simulink model "rcservo1"  (Simulink 7.8)
settings: Solver=ode45  StartTime=0.0  StopTime=10.0  RelTol=1e-3
values from neighbouring files (symbols this model uses):
  atemp = 1e9    (= 1000000000)    [ncf4.m]
libraries: cstblocks x8, simulink x4
settings Model: Creator=kas1d  LastModifiedBy=fukawa
settings DebuggingCC: AlgebraicLoopMsg=none  SolverPrmCheckMsg=none  FcnCallInpInsideContextMsg=Use local settings  UnconnectedInputMsg=none  UnconnectedOutputMsg=none  UnconnectedLineMsg=none

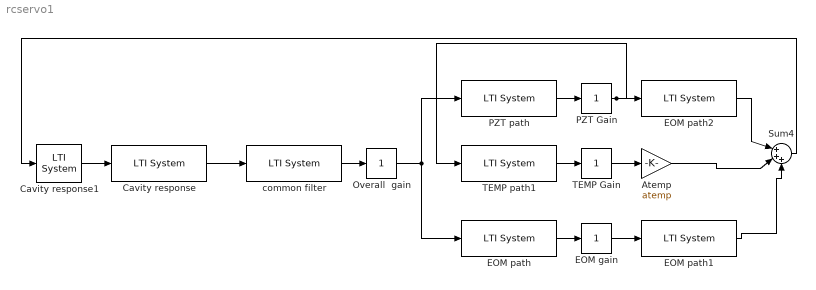
== system rcservo1 ==
  Atemp : Gain  Gain=atemp  SaturateOnIntegerOverflow=on  OutDataTypeStr=Inherit: Same as input  ParamDataTypeStr=Inherit: Same as input
  Cavity response : cstblocks/LTI System  sys=cavity  IC=[0]
  Cavity response1 : cstblocks/LTI System  sys=pmc  IC=[0]
  EOM gain : simulink/Math Operations/Slider Gain  low=0  gain=1  high=2
  EOM path : cstblocks/LTI System  sys=geom  IC=[0]
  EOM path1 : cstblocks/LTI System  sys=aeom  IC=[0]
  EOM path2 : cstblocks/LTI System  sys=apzt  IC=[0]
  Overall  gain : simulink/Math Operations/Slider Gain  low=-1  gain=1  high=2
  PZT Gain : simulink/Math Operations/Slider Gain  low=0  gain=1  high=2
  PZT path : cstblocks/LTI System  sys=gpzt  IC=[0]
  Sum4 : Sum  Inputs=|+++
  TEMP Gain : simulink/Math Operations/Slider Gain  low=0  gain=1  high=2
  TEMP path1 : cstblocks/LTI System  sys=gtemp  IC=[0]
  common filter : cstblocks/LTI System  sys=common  IC=[0]
  wires:
  PZT path/1 -> PZT Gain/1
  PZT Gain/1 -> TEMP path1/1, EOM path2/1
  TEMP Gain/1 -> Atemp/1
  Atemp/1 -> Sum4/2
  TEMP path1/1 -> TEMP Gain/1
  EOM path/1 -> EOM gain/1
  common filter/1 -> Overall  gain/1
  Overall  gain/1 -> PZT path/1, EOM path/1
  EOM gain/1 -> EOM path1/1
  EOM path1/1 -> Sum4/3
  Cavity response/1 -> common filter/1
  EOM path2/1 -> Sum4/1
  Sum4/1 -> Cavity response1/1
  Cavity response1/1 -> Cavity response/1
